simulink library "adi_ad9361_models"  (R2019b)
settings: Solver=VariableStepAuto  StartTime=0.0  StopTime=10.0  RelTol=1e-3
undefined symbols (not defined in the file): ad9361_preload, D, dBval, DCLeak_Matrix, designMultirateFIR, errordlg, fuzz_val, GainImb_Matrix, IP2_Matrix, IP3_Matrix, magnitude
libraries: simrfV2elements x20, simrfV2util1 x10, dsparch4 x8, simrfV2junction1 x8, simulink x8, dspmlti4 x6, ad9361_private x4, simulink_extras x2, dspsigattribs x2, simrfV2sources1 x2, simrfV2_lib x2, dspmathops x2
(part 1 of 2)
settings Model: Creator=gzucchel  LastModifiedBy=bhisma
settings SolverCC: MinimalZcImpactIntegration=on
settings DataIOCC: ReturnWorkspaceOutputs=off
settings DebuggingCC: PregeneratedLibrarySubsystemCodeDiagnostic=none  ArithmeticOperatorsInVariantConditions=warning
settings SFSimCC: SimUseLocalCustomCode=off  CustomCodeUndefinedFunction=UseInterfaceOnly
settings RTWCC: RTWUseLocalCustomCode=off
settings CodeAppCC: StateflowObjectComments=on

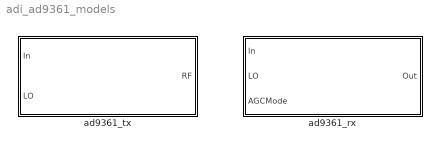
== system adi_ad9361_models ==
  ad9361_rx : Subsystem  LoadFcn=ad9361_preload(bdroot,'rx')  mask(ad9361_RX){TestSignal=Custom, LO=5200000000, RF=5200000000, Trf=5e-08/2, RF_BW=40, IQ_rate=40}
      mask prompts: TestSignal "Filter Configuration:"; LO "LO Frequency (Hz)"; RF "RF Center Frequency (Hz)"; Trf "Step Size RF Simulation (s)"; RF_BW "Input RF Bandwidth (MHz)"; IQ_rate "I/Q Sample Rate (MHz)"
      mask help: Model an Analog Devices ad9361 RF Receiver.
      mask init:
      | %load ad9361_rx_tables;
      | [ADIGainTable, ADIPhaseTable, ...
      |     DCLeak_Matrix, GainImb_Matrix, ...
      |     IP2_Matrix, IP3_Matrix] = ad9361_rx_gaintable(LO);
      | ad9361_rx_pars = ad9361_rx_initfcn(gcb,'Init');
      | ad9361_rx_pars = ad9361_rx_initfcn(gcb,'Build');
      mask Help:
      | Model an Analog Devices ad9361 RF Receiver. This model predicts thermal noise, spectral growth, LO carrier leakage and image signals, quantization noise in manual and slow attack control mode.
      | 
      | To change the automatic gain control mode, toggle the manual switch between manual mode and slow-attack control mode under the receiver mask. For manual mode, directly specify the index of the gain table in the constant block "manual index".
      | 
      | For signals with LTE 5MHz, LTE 10 MHz and LTE 20 MHz characteristics, the default configurations recommended by Analog Devices are directly available.
      | 
      | The filters are programmable. Use the Analog Devices Wizard App to custom design Filters. Select the option Custom in the Filter Configuration menu and click Design Filter button. The Filter Design app will open automatically. Make sure a receiver filter is designed instead of a transmitter filter. After designing the filter, click the button Export to Workspace in the App. The custom filter design is saved in the model set up. Next time a simulation is setup with custom filter configuration, the latest filter design is used.
      | 
      | Make sure that the input signal sample time and the expected step size of the RF simulation are the same. In case of a mismatch, an error is generated.
      mask TypeOptions TestSignal: 5MHz LTE | 10MHz LTE | 20MHz LTE | Custom
      mask Callback TestSignal:
      | % Set Mask visibilites and enables
      | ad9361_rx_mask_callbacks(gcb,'TestSignal')
      mask Callback Trf:
      | % block = gcb;
      | % p = Simulink.Mask.get(block);
      | % tmp = num2str(1/eval(get_param(gcb,'Trf'))/1e6,6);
      | % p.Parameters(5).Value = tmp;
      | set_param(gcb,'RF_BW',num2str(1/eval(get_param(gcb,'Trf'))/1e6,6));
      mask DialogControl ParameterGroupVar Prompt: ad9361 Receiver
      mask DialogControl Control2 Prompt: SpacerDesign
      mask DialogControl DesignFilter Prompt: Design Filter
      mask DialogControl DesignFilter Callback: ad9361_rx_initfcn(gcb,'DesignFilter');
      mask Display: text(0.5,0.5,'ad9361_RX','horizontalAlignment','center');
  ad9361_tx : Subsystem  LoadFcn=ad9361_preload(bdroot,'tx')  mask(ad9361_TX){TestSignal=5MHz LTE, LOFreq=2e9, Att=0, IQ_rate=7.68, RF_BW=122.88}
      mask prompts: TestSignal "Filter Configuration:"; LOFreq "LO Frequency (Hz)"; Att "Attenuation (dB)"; IQ_rate "I/Q Sample Rate (MHz)"; RF_BW "RF Bandwidth (MHz)"
      mask help: Model an Analog Devices ad9361 RF Transmitter.
      mask init:
      | ad9361_tx_pars = ad9361_tx_initfcn(gcb,'Init');
      | ad9361_tx_pars = ad9361_tx_initfcn(gcb,'Build');
      mask Help:
      | Model an Analog Devices ad9361 RF Transmitter. This predicts thermal noise, phase noise, spectral growth, LO carrier leakage and image signals.
      | 
      | To change the attenuation value, modify the constant value in Attenuation block under the Transmitter mask. Transmitter attenuation is tunable between 0 to 80dB in steps of 0.25dB.
      | 
      | For signals with LTE 5MHz, LTE 10 MHz and LTE 20 MHz characteristics, the default configurations recommended by Analog Devices are directly available.
      | 
      | The filters are programmable. Use the Analog Devices Wizard App to custom design Filters. Select the option Custom in the Filter Configuration menu and click Design Filter button. The Filter Design App will open automatically. Make sure a transmitter filter is designed instead of a receiver filter. After designing the filter, click the button Export to Workspace in the App. The custom filter design is saved in the model set up. Next time a simulation is setup with custom filter configuration, the latest filter design is used.
      | 
      | Make sure that the input signal sample time and the expected signal sample time are the same. In case of a mismatch, an error is generated.
      mask TypeOptions TestSignal: 5MHz LTE | 10MHz LTE | 20MHz LTE | Custom
      mask Callback TestSignal:
      | % Control DesignFilter visibility
      | ad9361_tx_mask_callbacks(gcb,'TestSignal')
      mask DialogControl ParameterGroupVar Prompt: ad9361 Transmitter
      mask DialogControl DesignFilter Prompt: Design Filter
      mask DialogControl DesignFilter Callback: [~] = ad9361_tx_initfcn(gcb,'DesignFilter');
      mask DialogControl Control3 Prompt: SpacerDesign
      mask Display: text(0.5,0.5,'ad9361_TX','horizontalAlignment','center');

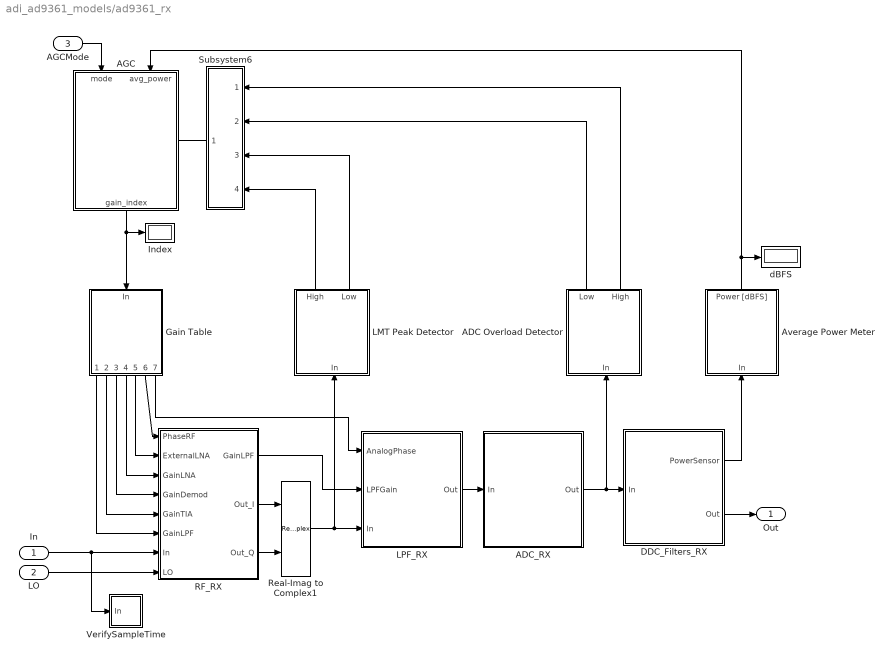
== system adi_ad9361_models/ad9361_rx ==
  In : Inport
  LO : Inport  Port=2
  AGCMode : Inport  Port=3
  ADC Overload Detector : Subsystem  mask{Ncycles=4, Lthreshold=47, Hthreshold=58}
      mask prompts: Ncycles "Number of Integration Cycles"; Lthreshold "Low Threshold"; Hthreshold "High Threshold"
      mask DialogControl DescGroupVar Prompt: ADC Overload Detector
  ADC_RX : Subsystem
  AGC : Stateflow chart  TreatAsAtomicUnit=on  mask{T=1, PeakOverLoadWait=1, SettlingDelay=32, FIR_Ts=ad9361_rx_pars.Tadc*ad9361_rx_pars.HB_interp, LMT_G_dec_fast=2, ADC_G_dec_fast=2, AGC_G_dec_fast=1, AGC_G_dec_slow=1, AGC_G_inc_fast=1, AGC_G_inc_slow=1, ManualGainIndex=76, C=3072 %approx 0.2ms, N_LMT_H=10, N_LMT_L=10, N_ADC_H=10, N_ADC_L=10, PT_HH=-8, PT_H=-10, PT_L=-12, PT_LL=-15, AGC_lock_level=-10, Max_Increase=5, EnableIncrGain=1, EnableGainIncAfterLock=1, AGC_attack_delay=10, EnergyDetectCount=32, IncrTime=5, LowPower=-13, PostLockStepSize=1, PowerMeasDuration=64, GainReset=No Gain Change, GainOffset=5, EnergyLost=1, StrongerSignalThreshold=10, GainLockExitCount=8, Overrange=8}
      mask prompts: T "Extra delay margin [us]"; PeakOverLoadWait "Peak Overload Wait Time [cycles]"; SettlingDelay "Settling Delay Power Meter [cycles]"; FIR_Ts "FIR Input Clock Time"; LMT_G_dec_fast "LMT peak large decrement"; ADC_G_dec_fast "ADC peak large decrement"; AGC_G_dec_fast "Average Power large decrement"; AGC_G_dec_slow "Average Power small decrement"; AGC_G_inc_fast "Average Power large increment"; AGC_G_inc_slow "Average Power small increment"; ManualGainIndex "Gain Index"; C "Gain Update Counter [cycles]"; N_LMT_H "LMT Upper Count"; N_LMT_L "LMT Lower Count"; N_ADC_H "ADC Upper Count"; N_ADC_L "ADC Lower Count"; PT_HH "Outer Threshold High [dBFS]"; PT_H "Inner Threshold High [dBFS]"; PT_L "Inner Threshold Low [dBFS]"; PT_LL "Outer Threshold Low [dBFS]"; AGC_lock_level "AGC Lock Level [dBFS]"; Max_Increase "AGC Lock Level Max Increase [Index]"; EnableIncrGain "Enable Gain Increment [0/1]"; EnableGainIncAfterLock "Enable Gain Increment After Gain Lock [0/1]"; AGC_attack_delay "Attack delay [us]"; EnergyDetectCount "Energy Detect Count [cycles]"; IncrTime "Increment Time [cycles]"; LowPower "Low Power Threshold"; PostLockStepSize "Post Lock Level Step Size [Index]"; PowerMeasDuration "Power Measurement Duration - State 5 [cycles]"; GainReset "Gain Index When Reset"; GainOffset "Optimize Gain Offset"; EnergyLost "Energy Lost Level [dB]"; StrongerSignalThreshold "Stronger Signal Threshold [dB]"; GainLockExitCount "Gain Lock Exit Count [cycles]"; Overrange "Overrange Count [Events]"
      mask init:
      | EnergyDetectCount = EnergyDetectCount*FIR_Ts;
      | C = C*FIR_Ts;
      | SettlingDelay = SettlingDelay*FIR_Ts;
      | PeakOverLoadWait = PeakOverLoadWait*FIR_Ts;
      | PowerMeasDuration = PowerMeasDuration*FIR_Ts;
      | IncrTime = IncrTime*FIR_Ts;
      | 
      | tmp = get_param(gcb,'parent');
      | n = get_param([tmp, '/Average Power Meter'], 'Ncycles');
      | DecPowerMeasDuration = str2num(n)*FIR_Ts;
  Average Power Meter : Subsystem  mask{Ncycles=64}
      mask prompts: Ncycles "Number of Integration Cycles"
      mask DialogControl DescGroupVar Prompt: Average Power Meter
  DDC_Filters_RX : Subsystem
  Gain Table : Subsystem
  "Index " : Display
  LMT Peak Detector : Subsystem  mask{HThreshold=800, LThreshold=704}
      mask prompts: HThreshold "High Threshold [mV]"; LThreshold "Low Threshold [mV]"
      mask DialogControl DescGroupVar Prompt: LMT Peak Detector
  LPF_RX : Subsystem
  RF_RX : Subsystem  mask{RF=RF, LO=LO, Tstep=Trf}
      mask prompts: RF "Center Frequency [Hz]"; LO "LO Frequency [Hz]"; Tstep "Sample Time [s]"
      mask init:
      | freq = [0.8e9, 2.4e9, 5.5e9];
      | nf   = [2,     3,     3.8];
      | NF   = interp1(freq, nf, LO,'linear','extrap');
      | 
      | if length(unique([RF LO])) == 2
      |     HB = [3 1];
      | else
      |     HB = 3;
      | end
      mask DialogControl DescGroupVar Prompt: ad9361 Receiver RF Front End
  Real-Imag to Complex1 : RealImagToComplex
  Subsystem6 : Subsystem  mask{NCyclesADC=4}
      mask prompts: NCyclesADC "ADC Integration Cycles"
  VerifySampleTime : Subsystem
  dBFS : Display
  Out : Outport  VectorParamsAs1DForOutWhenUnconnected=off
  wires:
  LO/1 -> RF_RX/8(LO)
  Gain Table/7(Analog phase) -> LPF_RX/1(AnalogPhase)
  ADC_RX/1(Out) -> DDC_Filters_RX/1(In), ADC Overload Detector/1(In)
  AGC/1(gain_index) -> "Index "/1, Gain Table/1(In)
  Average Power Meter/1(Power [dBFS]) -> AGC/2(avg_power), dBFS/1
  AGCMode/1 -> AGC/1(mode)
  Gain Table/5(External LNA) -> RF_RX/2(ExternalLNA)
  RF_RX/1("GainLPF ") -> LPF_RX/2(LPFGain)
  Subsystem6/1(Peak) -> AGC/Trigger
  In/1 -> VerifySampleTime/1(In), RF_RX/7(In)
  DDC_Filters_RX/2(Out) -> Out/1
  ADC Overload Detector/1(Low) -> Subsystem6/2(ADC_L)
  LMT Peak Detector/1(High) -> Subsystem6/4(LMT_H)
  ADC Overload Detector/2(High) -> Subsystem6/1(ADC_H)
  DDC_Filters_RX/1(PowerSensor) -> Average Power Meter/1(In)
  Gain Table/1(lpf) -> RF_RX/6(GainLPF)
  LMT Peak Detector/2(Low) -> Subsystem6/3(LMT_L)
  LPF_RX/1(Out) -> ADC_RX/1(In)
  Gain Table/4(lna) -> RF_RX/3(GainLNA)
  Gain Table/3(demod) -> RF_RX/4(GainDemod)
  Gain Table/2(tia) -> RF_RX/5(GainTIA)
  Real-Imag to Complex1/1 -> LPF_RX/3(In), LMT Peak Detector/1(In)
  RF_RX/3(Out_Q) -> Real-Imag to Complex1/2
  RF_RX/2(Out_I) -> Real-Imag to Complex1/1
  Gain Table/6(RF phase) -> RF_RX/1(PhaseRF)

== system adi_ad9361_models/ad9361_tx ==
  In : Inport
  LO : Inport  Port=2
  Analog_Filters_TX : Subsystem
  Attenuation : Constant  Value=Att
  DUC_Filters_TX : Subsystem
  RF_TX : Subsystem  mask{RF=LOFreq, Tstep=ad9361_tx_pars.Tduc}
      mask prompts: RF "Center Frequency (Hz)"; Tstep "Sample Time (s)"
      mask init:
      | Gain = interp1([800e6, 2.4e9, 5.5e9], [0, 0, -1]+8.3, RF, 'linear', 'extrap');
      | 
      | % Output referred IP3
      | oip3_800MHz = [23, 25, 10, 10];
      | oip3_2p4GHz = [19, 18,  6,  6];
      | oip3_5p5GHz = [17, 13,  2,  2];
      | Att_ip3     = [0 4 20 80];
      | if RF < 1.6e9
      |     OIP3v = oip3_800MHz;
      | elseif RF < 4e9
      |     OIP3v = oip3_2p4GHz;
      | else
      |     OIP3v = oip3_5p5GHz;
      | end
      | % Attenuation measurement data (dB)
      | Attdata  = [0  10  20  30  40  50   60   70   80];
      | % LO carrier leakage (dBm)
      | LO_leak  = ([-58 -52 -60 -71 -81 -82 -101 -102 -100]-Gain-6)/10;
      | % Gain imbalance (dBc)
      | Gain_imb = [-55.5 -66.2 -53.5 -57.5 -44.5 -46.3 -54.2 -46.1 -34.3]/20;
      | % Thermal noise floor (dBm/Hz)
      | NF       = interp1([800e6, 2.4e9, 5.5e9], [17, 18, 22.5], RF, 'linear', 'extrap');
      | 
      | set_param([gcb '/Configuration'], 'AddNoise','on');
      mask DialogControl Container1 Prompt: ad9361 Transmitter RF Front End
  VerifySampleTime : Subsystem
  RF : Outport  VectorParamsAs1DForOutWhenUnconnected=off
  wires:
  LO/1 -> RF_TX/4(LO)
  RF_TX/1(Out) -> RF/1
  DUC_Filters_TX/1(Out) -> Analog_Filters_TX/1(In)
  Attenuation/1 -> RF_TX/3(Attenuation)
  In/1 -> DUC_Filters_TX/1(In), VerifySampleTime/1(In)
  Analog_Filters_TX/2(Imaginary) -> RF_TX/2(In_Q)
  Analog_Filters_TX/1(Real) -> RF_TX/1(In_I)

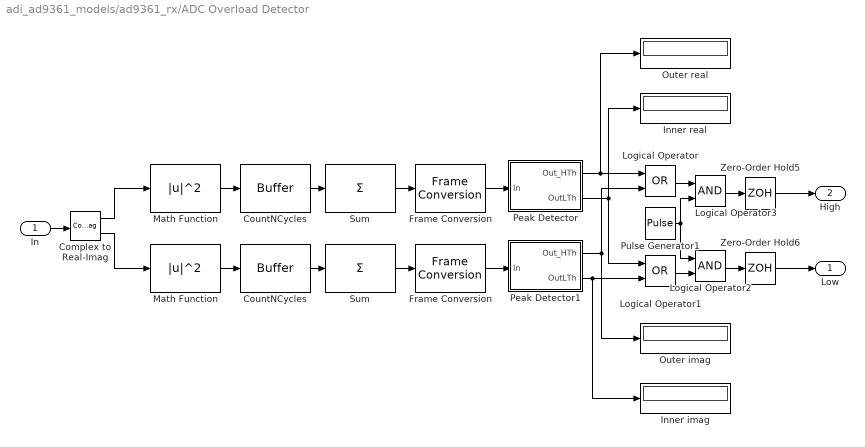
== system adi_ad9361_models/ad9361_rx/ADC Overload Detector ==
  In : Inport
  Complex to Real-Imag : ComplexToRealImag
  CountNCycles : Buffer  N=Ncycles
  "CountNCycles " : Buffer  N=Ncycles
  Frame Conversion : FrameConversion  OutFrame=Sample-based
  "Frame Conversion " : FrameConversion  OutFrame=Sample-based
  Inner imag : Display
  Inner real : Display
  Logical Operator : Logic  Operator=OR  AllPortsSameDT=off  OutDataTypeStr=boolean
  Logical Operator1 : Logic  Operator=OR  AllPortsSameDT=off  OutDataTypeStr=boolean
  Logical Operator2 : Logic  AllPortsSameDT=off  OutDataTypeStr=boolean
  Logical Operator3 : Logic  AllPortsSameDT=off  OutDataTypeStr=boolean
  Math Function : Math  Operator=magnitude^2  SaturateOnIntegerOverflow=on
  "Math Function " : Math  Operator=magnitude^2  SaturateOnIntegerOverflow=on
  Outer imag : Display
  Outer real : Display
  Peak Detector : Subsystem  mask{HThreshold=Hthreshold, LThreshold=Lthreshold}
      mask prompts: HThreshold "High Threshold (bit string) <4:0>"; LThreshold "Low Threshold (bit string) <4:0>"
  Peak Detector1 : Subsystem  mask{HThreshold=Hthreshold, LThreshold=Lthreshold}
      mask prompts: HThreshold "High Threshold (bit string) <4:0>"; LThreshold "Low Threshold (bit string) <4:0>"
  Pulse Generator1 : DiscretePulseGenerator  SampleTime=ad9361_rx_pars.Tadc*Ncycles
  Sum : Sum  Inputs=+
  "Sum " : Sum  Inputs=+
  Zero-Order Hold5 : ZeroOrderHold  SampleTime=Trf
  Zero-Order Hold6 : ZeroOrderHold  SampleTime=Trf
  Low : Outport  VectorParamsAs1DForOutWhenUnconnected=off
  High : Outport  Port=2  VectorParamsAs1DForOutWhenUnconnected=off
  wires:
  Zero-Order Hold6/1 -> Low/1
  Zero-Order Hold5/1 -> High/1
  Pulse Generator1/1 -> Logical Operator3/2, Logical Operator2/1
  Logical Operator3/1 -> Zero-Order Hold5/1
  Logical Operator1/1 -> Logical Operator2/2
  Logical Operator2/1 -> Zero-Order Hold6/1
  Logical Operator/1 -> Logical Operator3/1
  Complex to Real-Imag/2 -> "Math Function "/1
  Complex to Real-Imag/1 -> Math Function/1
  Peak Detector1/2(OutLTh) -> Logical Operator1/2, Inner imag/1
  Peak Detector1/1(Out_HTh) -> Outer imag/1, Logical Operator/2
  Peak Detector/1(Out_HTh) -> Logical Operator/1, Outer real/1
  Peak Detector/2(OutLTh) -> Inner real/1, Logical Operator1/1
  "Frame Conversion "/1 -> Peak Detector1/1(In)
  "Sum "/1 -> "Frame Conversion "/1
  "CountNCycles "/1 -> "Sum "/1
  "Math Function "/1 -> "CountNCycles "/1
  In/1 -> Complex to Real-Imag/1
  Frame Conversion/1 -> Peak Detector/1(In)
  Sum/1 -> Frame Conversion/1
  CountNCycles/1 -> Sum/1
  Math Function/1 -> CountNCycles/1

== system adi_ad9361_models/ad9361_rx/ADC_RX ==
  In : Inport
  ADC_I : Subsystem
  ADC_Q : Subsystem
  Complex to Real-Imag1 : ComplexToRealImag
  Real-Imag to Complex : RealImagToComplex
  Out : Outport  VectorParamsAs1DForOutWhenUnconnected=off
  wires:
  ADC_Q/1(Out) -> Real-Imag to Complex/2
  ADC_I/1(Out) -> Real-Imag to Complex/1
  Real-Imag to Complex/1 -> Out/1
  In/1 -> Complex to Real-Imag1/1
  Complex to Real-Imag1/2 -> ADC_Q/1(In)
  Complex to Real-Imag1/1 -> ADC_I/1(In)

== system adi_ad9361_models/ad9361_rx/Average Power Meter ==
  In : Inport
  Max saturation power dBm : Constant  Value=20*log10(4)+30
  Quantizer : Quantizer
  RMS : Subsystem
  Saturation : Saturate  UpperLimit=0  LowerLimit=-63.5
  Subtract : Sum  Inputs=+-
  dB Conversion : Subsystem  mask(dB Conversion){dBtype=dBm, intype=Amplitude, R=1, fuzz=on}
      mask prompts: dBtype "Convert to:"; intype "Input signal:"; R "Load resistance (ohms):"; fuzz "Add eps to input to protect against  "log(0) = -inf""
      mask help: Convert input of watts or volts to decibels. Voltage inputs are first converted to power relative to the specified load resistance, where P = (V^2)/R. When converting to dB, the reference power is 1 W. When converting to dBm, the reference power is 1 mW.
      mask init:
      | [str fuzz_val dBval] = dspblkdb2('init');
      | dspblkdb2('checkparam');
      | dspblkdb2('update');
      mask Help: eval('blocksethelp');
      mask TypeOptions dBtype: dB | dBm
      mask Callback dBtype: dspblkdb2
      mask TypeOptions intype: Power | Amplitude
      mask Callback intype: dspblkdb2
      mask Display: disp(str)
  Power [dBFS] : Outport  VectorParamsAs1DForOutWhenUnconnected=off
  wires:
  Saturation/1 -> Power [dBFS]/1
  RMS/1(Out) -> dB Conversion/1(in)
  In/1 -> RMS/1(In)
  dB Conversion/1(out) -> Subtract/1
  Quantizer/1 -> Saturation/1
  Subtract/1 -> Quantizer/1
  Max saturation power dBm/1 -> Subtract/2

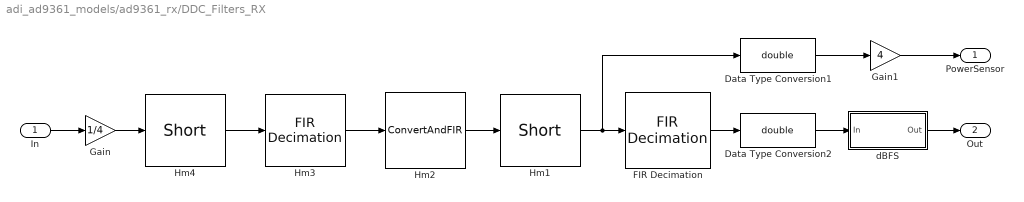
== system adi_ad9361_models/ad9361_rx/DDC_Filters_RX ==
  In : Inport
  Data Type Conversion1 : DataTypeConversion  OutDataTypeStr=double
  Data Type Conversion2 : DataTypeConversion  OutDataTypeStr=double
  FIR Decimation : dspmlti4/FIR Decimation  FilterSource=Filter object  h=fir1(35,0.4)  D=2  filtStruct=Direct form  FilterObject=ad9361_rx_pars.Hmd_rx  framing=Allow multirate processing  inputOffset=0  outputBufInitCond=0  roundingMode=Floor  overflowMode=off  firstCoeffDataTypeStr=Inherit: Same word length as input  firstCoeffMin=[]  firstCoeffMax=[]  firstCoeffLastDataTypeStr=Inherit: Same word length as input  outputDataTypeStr=Inherit: Same as accumulator  outputMin=[]  outputMax=[]  outputLastDataTypeStr=Inherit: Same as accumulator
  Gain : Gain  Gain=1/4
  Gain1 : Gain  Gain=4
  Hm1 : ad9361_private/Short  SystemSampleTime=-1  VariantControl=ad9361_tx_hm1Filt==0
      settings: SourceProductName=RF Blockset Models for Analog Devices RF Transceivers  SourceProductBaseCode=SIM_RF_TRANS
  Hm2 : ad9361_private/ConvertAndFIR  DataTypeOut=fixdt(1,16,14)  FilterObj=ad9361_rx_pars.Hm2_rx
      settings: SourceProductName=RF Blockset Models for Analog Devices RF Transceivers  SourceProductBaseCode=SIM_RF_TRANS
  Hm3 : dspmlti4/FIR Decimation  FilterSource=Filter object  h=designMultirateFIR(1,2)  D=2  filtStruct=Direct form  FilterObject=ad9361_rx_pars.Hm3_rx  framing=Enforce single-rate processing  inputOffset=0  outputBufInitCond=0  roundingMode=Floor  overflowMode=off  firstCoeffDataTypeStr=Inherit: Same word length as input  firstCoeffMin=[]  firstCoeffMax=[]  firstCoeffLastDataTypeStr=Inherit: Same word length as input  outputDataTypeStr=Inherit: Same as accumulator  outputMin=[]  outputMax=[]  outputLastDataTypeStr=Inherit: Same as accumulator
  Hm4 : ad9361_private/Short  SystemSampleTime=-1  VariantControl=ad9361_tx_hm1Filt==0
      settings: SourceProductName=RF Blockset Models for Analog Devices RF Transceivers  SourceProductBaseCode=SIM_RF_TRANS
  dBFS : Subsystem
  PowerSensor : Outport  VectorParamsAs1DForOutWhenUnconnected=off
  Out : Outport  Port=2  VectorParamsAs1DForOutWhenUnconnected=off
  wires:
  dBFS/1(Out) -> Out/1
  Data Type Conversion2/1 -> dBFS/1(In)
  Hm1/1 -> Data Type Conversion1/1, FIR Decimation/1
  Gain1/1 -> PowerSensor/1
  Data Type Conversion1/1 -> Gain1/1
  Gain/1 -> Hm4/1
  FIR Decimation/1 -> Data Type Conversion2/1
  Hm2/1 -> Hm1/1
  Hm3/1 -> Hm2/1
  Hm4/1 -> Hm3/1
  In/1 -> Gain/1

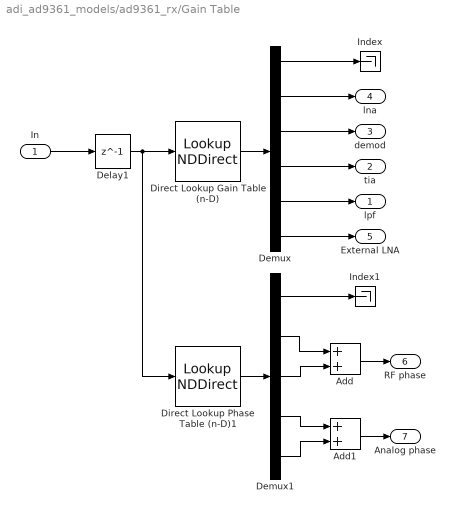
== system adi_ad9361_models/ad9361_rx/Gain Table ==
  In : Inport
  Add : Sum
  Add1 : Sum
  Delay1 : Delay  DelayLength=1  InitialCondition=76  SampleTime=Trf
  Demux : Demux  Outputs=6
  Demux1 : Demux  Outputs=5
  Direct Lookup Gain Table (n-D) : LookupNDDirect  InputsSelectThisObjectFromTable=Vector  Table=ADIGainTable'
  Direct Lookup Phase Table (n-D)1 : LookupNDDirect  InputsSelectThisObjectFromTable=Vector  Table=ADIPhaseTable'
  Index : Terminator
  Index1 : Terminator
  lpf : Outport  VectorParamsAs1DForOutWhenUnconnected=off
  tia : Outport  Port=2  VectorParamsAs1DForOutWhenUnconnected=off
  demod : Outport  Port=3  VectorParamsAs1DForOutWhenUnconnected=off
  lna : Outport  Port=4  VectorParamsAs1DForOutWhenUnconnected=off
  External LNA : Outport  Port=5  VectorParamsAs1DForOutWhenUnconnected=off
  RF phase : Outport  Port=6  VectorParamsAs1DForOutWhenUnconnected=off
  Analog phase : Outport  Port=7  VectorParamsAs1DForOutWhenUnconnected=off
  wires:
  Add1/1 -> Analog phase/1
  Add/1 -> RF phase/1
  Demux1/5 -> Add1/2
  Demux1/4 -> Add1/1
  Demux1/3 -> Add/2
  Demux1/2 -> Add/1
  Demux1/1 -> Index1/1
  Direct Lookup Phase Table (n-D)1/1 -> Demux1/1
  Demux/1 -> Index/1
  Demux/6 -> External LNA/1
  Direct Lookup Gain Table (n-D)/1 -> Demux/1
  Delay1/1 -> Direct Lookup Gain Table (n-D)/1, Direct Lookup Phase Table (n-D)1/1
  In/1 -> Delay1/1
  Demux/5 -> lpf/1
  Demux/4 -> tia/1
  Demux/2 -> lna/1
  Demux/3 -> demod/1

== system adi_ad9361_models/ad9361_rx/LMT Peak Detector ==
  In : Inport
  Abs : Abs
  HTh : Constant  Value=HThreshold*1e-3
  "High " : Display
  HighThreshold : RelationalOperator  OutDataTypeStr=boolean  RndMeth=Nearest
  LTh : Constant  Value=LThreshold*1e-3
  Logical Operator : Logic  AllPortsSameDT=off  OutDataTypeStr=boolean
  Logical Operator1 : Logic  AllPortsSameDT=off  OutDataTypeStr=boolean
  "Low " : Display
  LowThreshold : RelationalOperator  OutDataTypeStr=boolean  RndMeth=Nearest
  Pulse Generator2 : DiscretePulseGenerator  SampleTime=Trf
  High : Outport  SampleTime=Trf  VectorParamsAs1DForOutWhenUnconnected=off
  Low : Outport  Port=2  SampleTime=Trf  VectorParamsAs1DForOutWhenUnconnected=off
  wires:
  Logical Operator/1 -> Low/1
  Logical Operator1/1 -> High/1
  Pulse Generator2/1 -> Logical Operator/1, Logical Operator1/2
  LowThreshold/1 -> "Low "/1, Logical Operator/2
  HighThreshold/1 -> "High "/1, Logical Operator1/1
  In/1 -> Abs/1
  HTh/1 -> HighThreshold/2
  Abs/1 -> LowThreshold/1, HighThreshold/1
  LTh/1 -> LowThreshold/2

== system adi_ad9361_models/ad9361_rx/LPF_RX ==
  AnalogPhase : Inport
  LPFGain : Inport  Port=2
  In : Inport  Port=3
  Complex Phase Shift : commutil2/Complex Phase Shift
      settings: SourceProductName=Communications Toolbox  SourceProductBaseCode=CM
  Complex to Real-Imag : ComplexToRealImag
  Gain : Product
  LPF_I : dsparch4/Analog Filter Design  method=Butterworth  filttype=Lowpass  N=3  Wlo=1.4*ad9361_rx_pars.Fpass*2*pi  Whi=80  Rp=2  Rs=40
  "LPF_Q " : dsparch4/Analog Filter Design  method=Butterworth  filttype=Lowpass  N=3  Wlo=1.4*ad9361_rx_pars.Fpass*2*pi  Whi=80  Rp=2  Rs=40
  Phase[deg] : Display
  Real-Imag to Complex1 : RealImagToComplex
  ToRadians : Gain  Gain=pi/180
  dB2lin : Subsystem
  Out : Outport  VectorParamsAs1DForOutWhenUnconnected=off
  wires:
  ToRadians/1 -> Complex Phase Shift/2
  AnalogPhase/1 -> ToRadians/1, Phase[deg]/1
  In/1 -> Complex Phase Shift/1
  Complex to Real-Imag/2 -> "LPF_Q "/1
  LPF_I/1 -> Real-Imag to Complex1/1
  "LPF_Q "/1 -> Real-Imag to Complex1/2
  dB2lin/1(Out) -> Gain/1
  Gain/1 -> Complex to Real-Imag/1
  LPFGain/1 -> dB2lin/1(In)
  Complex Phase Shift/1 -> Gain/2
  Real-Imag to Complex1/1 -> Out/1
  Complex to Real-Imag/1 -> LPF_I/1

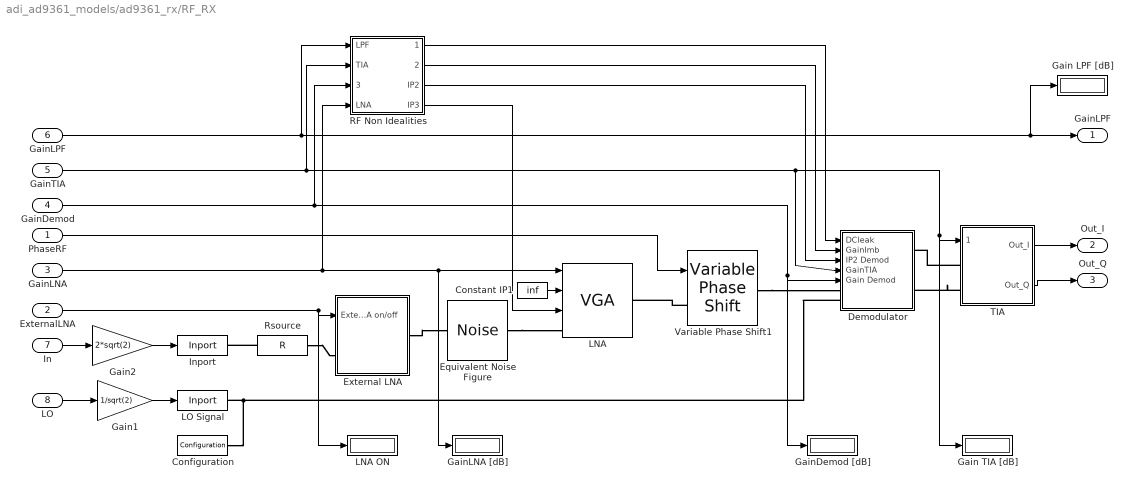
== system adi_ad9361_models/ad9361_rx/RF_RX ==
  PhaseRF : Inport
  ExternalLNA : Inport  Port=2
  GainLNA : Inport  Port=3
  GainDemod : Inport  Port=4
  GainTIA : Inport  Port=5
  GainLPF : Inport  Port=6
  In : Inport  Port=7
  LO : Inport  Port=8
  Configuration : simrfV2util1/Configuration  AutoFreq=off  Tones=unique([RF LO]) Hz  Harmonics=HB  NormalizeCarrierPower=on  SolverType=Auto  UseCCode=on  StepSize=Tstep s  AddNoise=on  defaultRNG=on  Seed=0  Temperature=290.0 K  SolverDelFlag=0  AbsTol=1e-6  RelTol=1e-3  MaxIter=10  ErrorEstimationType=2-norm over all variables  EnableInterpFilter=off  HiddenFIRfilterControllerParam=off  SmallSignalApprox=off  AllSimFreqs=on  SimFreqs=[] Hz  SimFreqsInternal=[]
      settings: SourceProductName=RF Blockset  SourceProductBaseCode=RB
  Constant IP1 : Constant  Value=inf
  Demodulator : Subsystem
  Equivalent Noise Figure : simrfV2sources1/Noise  SimulinkInputSignalType=Ideal voltage  NoiseType=White  NoisePSD=4*1.381e-23*290*50*10^(NF/10)  CarrierFreq=fc_RF Hz  AutoImpulseLength=on  ImpulseLength=1e-10 s  InternalGrounding=off
      settings: SourceProductName=RF Blockset  SourceProductBaseCode=RB
  External LNA : Subsystem
  Gain LPF [dB] : Display
  Gain TIA [dB] : Display
  Gain1 : Gain  Gain=1/sqrt(2)
  Gain2 : Gain  Gain=2*sqrt(2)
  GainDemod [dB] : Display
  GainLNA [dB] : Display
  Inport : simrfV2util1/Inport  SimulinkInputSignalType=Ideal voltage  CarrierFreq=RF Hz  ZS=0  InternalGrounding=on
      settings: SourceProductName=RF Blockset  SourceProductBaseCode=RB
  LNA : simrfV2elements/VGA  classname=vga  Zin=50  Zout=50  IO=Input  InternalGrounding=on
      settings: SourceProductName=RF Blockset  SourceProductBaseCode=RB
  LNA ON : Display
  LO Signal : simrfV2util1/Inport  SimulinkInputSignalType=Ideal voltage  CarrierFreq=LO Hz  ZS=0  InternalGrounding=on
      settings: SourceProductName=RF Blockset  SourceProductBaseCode=RB
  RF Non Idealities : Subsystem
  Rsource : simrfV2elements/R  classname=resistor  Resistance=50 Ohm  AddNoise=on
      settings: SourceProductName=RF Blockset  SourceProductBaseCode=RB
  TIA : Subsystem
  Variable Phase Shift1 : simrfV2elements/Variable Phase Shift  classname=varphase  PhaseShift_unit=deg  SparamZ0=50  InternalGrounding=on
      settings: SourceProductName=RF Blockset  SourceProductBaseCode=RB
  "GainLPF " : Outport  VectorParamsAs1DForOutWhenUnconnected=off
  Out_I : Outport  Port=2  VectorParamsAs1DForOutWhenUnconnected=off
  Out_Q : Outport  Port=3  VectorParamsAs1DForOutWhenUnconnected=off
  wires:
  Gain1/1 -> LO Signal/1
  LO/1 -> Gain1/1
  PhaseRF/1 -> Variable Phase Shift1/1
  TIA/2(Out_Q) -> Out_Q/1
  RF Non Idealities/2(GainImbalance) -> Demodulator/2(GainImb)
  ExternalLNA/1 -> External LNA/1(ExternalLNA on/off), LNA ON/1
  Constant IP1/1 -> LNA/2
  RF Non Idealities/4(IP3) -> LNA/3
  RF Non Idealities/3(IP2) -> Demodulator/3(IP2 Demod)
  RF Non Idealities/1(DCLeakage) -> Demodulator/1(DCleak)
  GainLNA/1 -> GainLNA [dB]/1, LNA/1, RF Non Idealities/4(LNA)
  GainDemod/1 -> RF Non Idealities/3(Demod), GainDemod [dB]/1, Demodulator/5(Gain Demod)
  GainTIA/1 -> RF Non Idealities/2(TIA), TIA/1(Gain TIA), Gain TIA [dB]/1, Demodulator/4(GainTIA)
  GainLPF/1 -> RF Non Idealities/1(LPF), Gain LPF [dB]/1, "GainLPF "/1
  TIA/1(Out_I) -> Out_I/1
  Gain2/1 -> Inport/1
  In/1 -> Gain2/1
  connections:
  Variable Phase Shift1/RConn1 -- Demodulator/LConn1
  Variable Phase Shift1/LConn1 -- LNA/RConn1
  Demodulator/LConn2 -- Configuration/LConn1 -- LO Signal/RConn1
  External LNA/RConn1 -- Equivalent Noise Figure/RConn1
  Rsource/LConn1 -- External LNA/LConn1
  TIA/LConn1 -- Demodulator/RConn1
  TIA/LConn2 -- Demodulator/RConn2
  Equivalent Noise Figure/LConn1 -- LNA/LConn1
  Rsource/RConn1 -- Inport/RConn1

== system adi_ad9361_models/ad9361_rx/Subsystem6 ==
  ADC_H : Inport
  ADC_L : Inport  Port=2
  LMT_L : Inport  Port=3
  LMT_H : Inport  Port=4
  Data Type Conversion : DataTypeConversion  OutDataTypeStr=boolean
  Logical Operator : Logic  Operator=OR  AllPortsSameDT=off  OutDataTypeStr=boolean
  Mux : Mux  Inputs=5
  Subsystem1 : Subsystem
  Wblk5 : Subsystem
  Wblk6 : Subsystem
  Wblk7 : Subsystem
  Peak : Outport  VectorParamsAs1DForOutWhenUnconnected=off
  wires:
  Mux/1 -> Peak/1
  LMT_H/1 -> Logical Operator/2, Mux/4, Wblk5/2(Sin)  "LMT_H"
  ADC_H/1 -> Wblk5/1(Win)
  ADC_L/1 -> Wblk6/1(Win)
  Data Type Conversion/1 -> Mux/5  "Event"
  Subsystem1/1(START) -> Data Type Conversion/1
  Wblk5/1(Wout) -> Logical Operator/1, Mux/1  "ADC_H"
  Wblk6/1(Wout) -> Mux/2  "ADC_L"
  Wblk7/1(Wout) -> Mux/3  "LMT_L"
  Logical Operator/1 -> Wblk6/2(Sin), Wblk7/2(Sin)
  LMT_L/1 -> Wblk7/1(Win)

== system adi_ad9361_models/ad9361_rx/VerifySampleTime ==
  In : Inport
  Abs : Abs
  Assertion : Assertion  AssertionFailFcn=errordlg('Test signal sample time and RF simulation step size are not consistent');
  Compare To Constant : simulink/Logic and Bit Operations/Compare To Constant  relop=<=  const=eps(1/Trf)  OutDataTypeStr=boolean
  Constant : Constant  Value=Trf
  Subtract : Sum  Inputs=+-
  Weighted Sample Time : SampleTimeMath  TsampMathOp=Ts Only
  wires:
  In/1 -> Weighted Sample Time/1
  Weighted Sample Time/1 -> Subtract/1
  Constant/1 -> Subtract/2
  Subtract/1 -> Abs/1
  Abs/1 -> Compare To Constant/1
  Compare To Constant/1 -> Assertion/1

== system adi_ad9361_models/ad9361_tx/Analog_Filters_TX ==
  In : Inport
  " AnalogFilter " : dsparch4/Analog Filter Design  method=Butterworth  filttype=Lowpass  N=3  Wlo=1.6*ad9361_tx_pars.Fpass*2*pi  Whi=80  Rp=2  Rs=40
  AnalogFilter : dsparch4/Analog Filter Design  method=Butterworth  filttype=Lowpass  N=3  Wlo=1.6*ad9361_tx_pars.Fpass*2*pi  Whi=80  Rp=2  Rs=40
  "AnalogFilter " : dsparch4/Analog Filter Design  method=Butterworth  filttype=Lowpass  N=1  Wlo=5*ad9361_tx_pars.Fpass*2*pi  Whi=80  Rp=2  Rs=40
  AnalogFilters : dsparch4/Analog Filter Design  method=Butterworth  filttype=Lowpass  N=1  Wlo=5*ad9361_tx_pars.Fpass*2*pi  Whi=80  Rp=2  Rs=40
  Complex to Real-Imag : ComplexToRealImag
  Real : Outport  VectorParamsAs1DForOutWhenUnconnected=off
  Imaginary : Outport  Port=2  VectorParamsAs1DForOutWhenUnconnected=off
  wires:
  AnalogFilters/1 -> Imaginary/1
  Complex to Real-Imag/1 -> AnalogFilter/1
  In/1 -> Complex to Real-Imag/1
  Complex to Real-Imag/2 -> " AnalogFilter "/1
  AnalogFilter/1 -> "AnalogFilter "/1
  " AnalogFilter "/1 -> AnalogFilters/1
  "AnalogFilter "/1 -> Real/1

== system adi_ad9361_models/ad9361_tx/DUC_Filters_TX ==
  In : Inport
  Add : Sum
  Band-Limited White Noise : simulink/Sources/Band-Limited White Noise  Cov=[0.1]  Ts=ad9361_tx_pars.Tduc  seed=[23341]
  Hm1 : dspmlti4/FIR Interpolation  FilterSource=Filter object  h=designMultirateFIR(3,1)  L=3  FilterObject=ad9361_tx_pars.Hm1_tx  framing=Enforce single-rate processing  outputBufInitCond=0  roundingMode=Floor  overflowMode=off  firstCoeffDataTypeStr=Inherit: Same word length as input  firstCoeffMin=[]  firstCoeffMax=[]  firstCoeffLastDataTypeStr=Inherit: Same word length as input  outputDataTypeStr=Inherit: Same as accumulator  outputMin=[]  outputMax=[]  outputLastDataTypeStr=Inherit: Same as accumulator
      settings: SourceProductName=DSP System Toolbox
  Hm2 : dspmlti4/FIR Interpolation  FilterSource=Filter object  h=designMultirateFIR(3,1)  L=3  FilterObject=ad9361_tx_pars.Hm2_tx  framing=Enforce single-rate processing  outputBufInitCond=0  roundingMode=Floor  overflowMode=off  firstCoeffDataTypeStr=Inherit: Same word length as input  firstCoeffMin=[]  firstCoeffMax=[]  firstCoeffLastDataTypeStr=Inherit: Same word length as input  outputDataTypeStr=Inherit: Same as accumulator  outputMin=[]  outputMax=[]  outputLastDataTypeStr=Inherit: Same as accumulator
      settings: SourceProductName=DSP System Toolbox
  Hm3 : dspmlti4/FIR Interpolation  FilterSource=Filter object  h=designMultirateFIR(3,1)  L=3  FilterObject=ad9361_tx_pars.Hm3_tx  framing=Enforce single-rate processing  outputBufInitCond=0  roundingMode=Floor  overflowMode=off  firstCoeffDataTypeStr=Inherit: Same word length as input  firstCoeffMin=[]  firstCoeffMax=[]  firstCoeffLastDataTypeStr=Inherit: Same word length as input  outputDataTypeStr=Inherit: Same as accumulator  outputMin=[]  outputMax=[]  outputLastDataTypeStr=Inherit: Same as accumulator
      settings: SourceProductName=DSP System Toolbox
  Hmd : dspmlti4/FIR Interpolation  FilterSource=Filter object  h=fir1(15,1/4)  L=3  FilterObject=ad9361_tx_pars.Hmd_tx  framing=Allow multirate processing  outputBufInitCond=0  roundingMode=Floor  overflowMode=off  firstCoeffDataTypeStr=Inherit: Same word length as input  firstCoeffMin=[]  firstCoeffMax=[]  firstCoeffLastDataTypeStr=Inherit: Same word length as input  outputDataTypeStr=Inherit: Same as accumulator  outputMin=[]  outputMax=[]  outputLastDataTypeStr=Inherit: Same as accumulator
      settings: SourceProductName=DSP System Toolbox
  NoiseFloor : dspmathops/dB Gain  dB=-130-20-8  intype=Amplitude
      settings: SourceProductName=DSP System Toolbox  SourceProductBaseCode=DS
  Short : ad9361_private/Short  SystemSampleTime=-1  VariantControl=ad9361_tx_hm1Filt==0
      settings: SourceProductName=RF Blockset Models for Analog Devices RF Transceivers  SourceProductBaseCode=SIM_RF_TRANS
  dB Gain : dspmathops/dB Gain  dB=log2(ad9361_tx_pars.BW_duc/ad9361_tx_pars.SamplingRate)*6  intype=Amplitude
      settings: SourceProductName=DSP System Toolbox  SourceProductBaseCode=DS
  Out : Outport  VectorParamsAs1DForOutWhenUnconnected=off
  wires:
  Hm2/1 -> Hm3/1
  Short/1 -> dB Gain/1
  NoiseFloor/1 -> Add/1
  Band-Limited White Noise/1 -> NoiseFloor/1
  Add/1 -> Out/1
  dB Gain/1 -> Add/2
  In/1 -> Hmd/1
  Hm3/1 -> Short/1
  Hm1/1 -> Hm2/1
  Hmd/1 -> Hm1/1

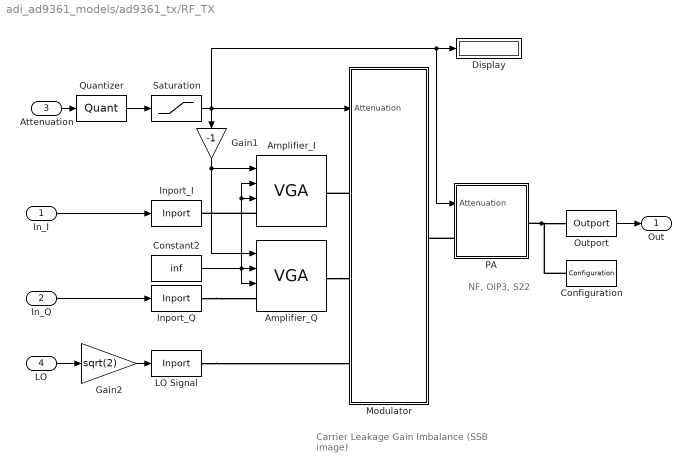
== system adi_ad9361_models/ad9361_tx/RF_TX ==
  note: Carrier Leakage
      | Gain Imbalance (SSB image)
  note: NF, OIP3, S22
  In_I : Inport
  In_Q : Inport  Port=2
  Attenuation : Inport  Port=3
  LO : Inport  Port=4
  Amplifier_I : simrfV2elements/VGA  classname=vga  Zin=50  Zout=50  IO=Output  InternalGrounding=on
      settings: SourceProductName=RF Blockset  SourceProductBaseCode=RB
  Amplifier_Q : simrfV2elements/VGA  classname=vga  Zin=50  Zout=50  IO=Output  InternalGrounding=on
      settings: SourceProductName=RF Blockset  SourceProductBaseCode=RB
  Configuration : simrfV2util1/Configuration  AutoFreq=off  Tones=RF Hz  Harmonics=3  NormalizeCarrierPower=on  SolverType=Auto  UseCCode=on  StepSize=Tstep s  AddNoise=on  defaultRNG=on  Seed=0  Temperature=290.0 K  SolverDelFlag=0  AbsTol=1e-6  RelTol=1e-3  MaxIter=10  ErrorEstimationType=2-norm over all variables  EnableInterpFilter=off  HiddenFIRfilterControllerParam=off  SmallSignalApprox=off  AllSimFreqs=on  SimFreqs=[] Hz  SimFreqsInternal=[]
      settings: SourceProductName=RF Blockset  SourceProductBaseCode=RB
  Constant2 : Constant  Value=inf
  Display : Display
      settings: Decimation=100
  Gain1 : Gain  Gain=-1
  Gain2 : Gain  Gain=sqrt(2)
  Inport_I : simrfV2util1/Inport  SimulinkInputSignalType=Power  CarrierFreq=0 Hz  ZS=50  InternalGrounding=on
      settings: SourceProductName=RF Blockset  SourceProductBaseCode=RB
  Inport_Q : simrfV2util1/Inport  SimulinkInputSignalType=Power  CarrierFreq=0 Hz  ZS=50  InternalGrounding=on
      settings: SourceProductName=RF Blockset  SourceProductBaseCode=RB
  LO Signal : simrfV2util1/Inport  SimulinkInputSignalType=Ideal voltage  CarrierFreq=LOFreq Hz  ZS=0  InternalGrounding=on
      settings: SourceProductName=RF Blockset  SourceProductBaseCode=RB
  Modulator : Subsystem
  Outport : simrfV2util1/Outport  SensorType=Power  OutputFormat=Complex Baseband  CarrierFreq=RF Hz  ZL=50  InternalGrounding=on  StepSize=-1 s  AutoStep=off
      settings: SourceProductName=RF Blockset  SourceProductBaseCode=RB
  PA : Subsystem
  Quantizer : Quantizer  QuantizationInterval=0.25
  Saturation : Saturate  UpperLimit=89.75  LowerLimit=0
  Out : Outport  VectorParamsAs1DForOutWhenUnconnected=off
  wires:
  Gain2/1 -> LO Signal/1
  LO/1 -> Gain2/1
  Gain1/1 -> Amplifier_Q/1, Amplifier_I/1
  Constant2/1 -> Amplifier_I/2, Amplifier_I/3, Amplifier_Q/2, Amplifier_Q/3
  Outport/1 -> Out/1
  Quantizer/1 -> Saturation/1
  Saturation/1 -> Display/1, PA/1(" Attenuation"), Modulator/1(Attenuation), Gain1/1
  Attenuation/1 -> Quantizer/1
  In_Q/1 -> Inport_Q/1
  In_I/1 -> Inport_I/1
  connections:
  LO Signal/RConn1 -- Modulator/LConn3
  Modulator/LConn1 -- Amplifier_I/RConn1
  PA/LConn1 -- Modulator/RConn1
  PA/RConn1 -- Outport/LConn1 -- Configuration/LConn1
  Amplifier_Q/RConn1 -- Modulator/LConn2
  Inport_Q/RConn1 -- Amplifier_Q/LConn1
  Amplifier_I/LConn1 -- Inport_I/RConn1

== system adi_ad9361_models/ad9361_tx/VerifySampleTime ==
  In : Inport
  Abs : Abs
  Assertion : Assertion  AssertionFailFcn=errordlg('Test signal sample time and I/Q sample rate are not consistent');
  Compare To Constant : simulink/Logic and Bit Operations/Compare To Constant  relop=<=  const=eps(1/ad9361_tx_pars.SamplingRate)*1e12  OutDataTypeStr=boolean
  Constant : Constant  Value=1/ad9361_tx_pars.SamplingRate
  Subtract : Sum  Inputs=+-
  Weighted Sample Time : SampleTimeMath  TsampMathOp=Ts Only
  wires:
  Compare To Constant/1 -> Assertion/1
  Subtract/1 -> Abs/1
  Constant/1 -> Subtract/2
  Weighted Sample Time/1 -> Subtract/1
  In/1 -> Weighted Sample Time/1
  Abs/1 -> Compare To Constant/1

== system adi_ad9361_models/ad9361_rx/ADC Overload Detector/Peak Detector ==
  In : Inport
  HTh : Constant  Value=Hthreshold  SampleTime=ad9361_rx_pars.Tadc*Ncycles
  HighThreshold : RelationalOperator  OutDataTypeStr=boolean  RndMeth=Nearest
  LTh : Constant  Value=Lthreshold  SampleTime=ad9361_rx_pars.Tadc*Ncycles
  LowThreshold : RelationalOperator  OutDataTypeStr=boolean  RndMeth=Nearest
  Out_HTh : Outport  VectorParamsAs1DForOutWhenUnconnected=off
  OutLTh : Outport  Port=2  VectorParamsAs1DForOutWhenUnconnected=off
  wires:
  HTh/1 -> HighThreshold/2
  In/1 -> LowThreshold/1, HighThreshold/1
  LTh/1 -> LowThreshold/2
  HighThreshold/1 -> Out_HTh/1
  LowThreshold/1 -> OutLTh/1

== system adi_ad9361_models/ad9361_rx/ADC Overload Detector/Peak Detector1 ==
  In : Inport
  HTh : Constant  Value=Hthreshold  SampleTime=ad9361_rx_pars.Tadc*Ncycles
  HighThreshold : RelationalOperator  OutDataTypeStr=boolean  RndMeth=Nearest
  LTh : Constant  Value=Lthreshold  SampleTime=ad9361_rx_pars.Tadc*Ncycles
  LowThreshold : RelationalOperator  OutDataTypeStr=boolean  RndMeth=Nearest
  Out_HTh : Outport  VectorParamsAs1DForOutWhenUnconnected=off
  OutLTh : Outport  Port=2  VectorParamsAs1DForOutWhenUnconnected=off
  wires:
  LowThreshold/1 -> OutLTh/1
  HighThreshold/1 -> Out_HTh/1
  LTh/1 -> LowThreshold/2
  In/1 -> HighThreshold/1, LowThreshold/1
  HTh/1 -> HighThreshold/2

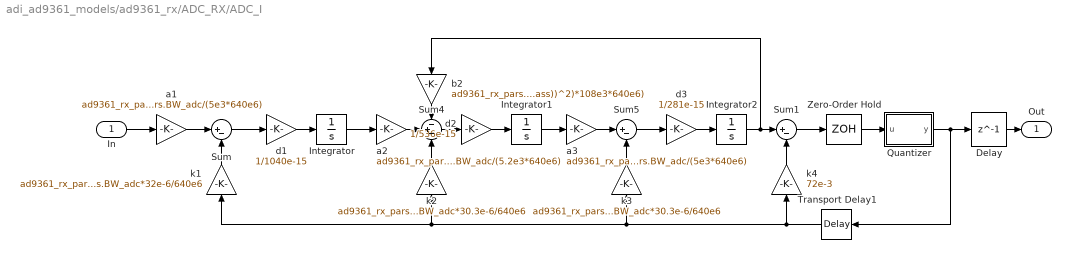
== system adi_ad9361_models/ad9361_rx/ADC_RX/ADC_I ==
  In : Inport
  Delay : Delay  DelayLength=1
  Integrator : Integrator  LimitOutput=on  UpperSaturationLimit=0.9  LowerSaturationLimit=-0.9
  Integrator1 : Integrator  LimitOutput=on  UpperSaturationLimit=0.9  LowerSaturationLimit=-0.9
  Integrator2 : Integrator  LimitOutput=on  UpperSaturationLimit=0.9  LowerSaturationLimit=-0.9
  Quantizer : Subsystem
  Sum : Sum  Inputs=|+-
  Sum1 : Sum  Inputs=|+-
  Sum4 : Sum  Inputs=-+-
  Sum5 : Sum  Inputs=|+-
  Transport Delay1 : TransportDelay  DelayTime=ad9361_rx_pars.Tadc/2
  Zero-Order Hold : ZeroOrderHold  SampleTime=ad9361_rx_pars.Tadc
  a1 : Gain  Gain=ad9361_rx_pars.BW_adc/(5e3*640e6)
  a2 : Gain  Gain=ad9361_rx_pars.BW_adc/(5.2e3*640e6)
  a3 : Gain  Gain=ad9361_rx_pars.BW_adc/(5e3*640e6)
  b2 : Gain  Gain=ad9361_rx_pars.BW_adc*1024/(4*((ad9361_rx_pars.BW_adc/(2*ad9361_rx_pars.Fpass))^2)*108e3*640e6)
  d1 : Gain  Gain=1/1040e-15
  d2 : Gain  Gain=1/536e-15
  d3 : Gain  Gain=1/281e-15
  k1 : Gain  Gain=ad9361_rx_pars.BW_adc*32e-6/640e6
  k2 : Gain  Gain=ad9361_rx_pars.BW_adc*30.3e-6/640e6
  k3 : Gain  Gain=ad9361_rx_pars.BW_adc*30.3e-6/640e6
  k4 : Gain  Gain=72e-3
  Out : Outport  VectorParamsAs1DForOutWhenUnconnected=off
  wires:
  Delay/1 -> Out/1
  Transport Delay1/1 -> k3/1, k2/1, k1/1, k4/1
  Quantizer/1(y) -> Delay/1, Transport Delay1/1
  k4/1 -> Sum1/2
  Sum1/1 -> Zero-Order Hold/1
  a3/1 -> Sum5/1
  b2/1 -> Sum4/1
  k3/1 -> Sum5/2
  k2/1 -> Sum4/3
  a2/1 -> Sum4/2
  Zero-Order Hold/1 -> Quantizer/1(u)
  Sum/1 -> d1/1
  Integrator/1 -> a2/1
  d1/1 -> Integrator/1
  Integrator1/1 -> a3/1
  d2/1 -> Integrator1/1
  Integrator2/1 -> b2/1, Sum1/1
  In/1 -> a1/1
  d3/1 -> Integrator2/1
  Sum4/1 -> d2/1
  Sum5/1 -> d3/1
  a1/1 -> Sum/1
  k1/1 -> Sum/2

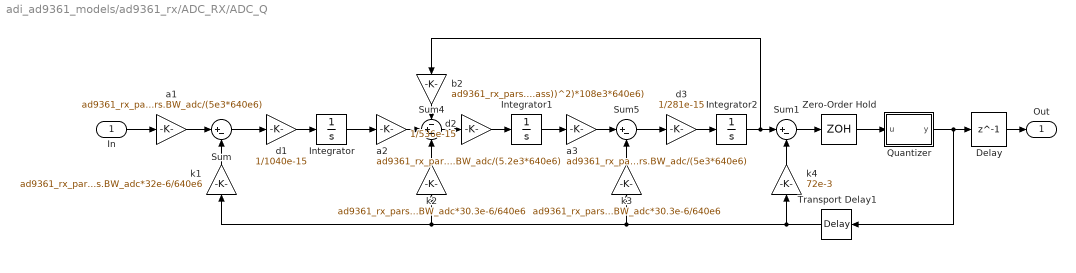
== system adi_ad9361_models/ad9361_rx/ADC_RX/ADC_Q ==
  In : Inport
  Delay : Delay  DelayLength=1
  Integrator : Integrator  LimitOutput=on  UpperSaturationLimit=0.9  LowerSaturationLimit=-0.9
  Integrator1 : Integrator  LimitOutput=on  UpperSaturationLimit=0.9  LowerSaturationLimit=-0.9
  Integrator2 : Integrator  LimitOutput=on  UpperSaturationLimit=0.9  LowerSaturationLimit=-0.9
  Quantizer : Subsystem
  Sum : Sum  Inputs=|+-
  Sum1 : Sum  Inputs=|+-
  Sum4 : Sum  Inputs=-+-
  Sum5 : Sum  Inputs=|+-
  Transport Delay1 : TransportDelay  DelayTime=ad9361_rx_pars.Tadc/2
  Zero-Order Hold : ZeroOrderHold  SampleTime=ad9361_rx_pars.Tadc
  a1 : Gain  Gain=ad9361_rx_pars.BW_adc/(5e3*640e6)
  a2 : Gain  Gain=ad9361_rx_pars.BW_adc/(5.2e3*640e6)
  a3 : Gain  Gain=ad9361_rx_pars.BW_adc/(5e3*640e6)
  b2 : Gain  Gain=ad9361_rx_pars.BW_adc*1024/(4*((ad9361_rx_pars.BW_adc/(2*ad9361_rx_pars.Fpass))^2)*108e3*640e6)
  d1 : Gain  Gain=1/1040e-15
  d2 : Gain  Gain=1/536e-15
  d3 : Gain  Gain=1/281e-15
  k1 : Gain  Gain=ad9361_rx_pars.BW_adc*32e-6/640e6
  k2 : Gain  Gain=ad9361_rx_pars.BW_adc*30.3e-6/640e6
  k3 : Gain  Gain=ad9361_rx_pars.BW_adc*30.3e-6/640e6
  k4 : Gain  Gain=72e-3
  Out : Outport  VectorParamsAs1DForOutWhenUnconnected=off
  wires:
  k1/1 -> Sum/2
  a1/1 -> Sum/1
  Sum5/1 -> d3/1
  Sum4/1 -> d2/1
  d3/1 -> Integrator2/1
  In/1 -> a1/1
  Integrator2/1 -> Sum1/1, b2/1
  d2/1 -> Integrator1/1
  Integrator1/1 -> a3/1
  d1/1 -> Integrator/1
  Integrator/1 -> a2/1
  Sum/1 -> d1/1
  Zero-Order Hold/1 -> Quantizer/1(u)
  a2/1 -> Sum4/2
  k2/1 -> Sum4/3
  k3/1 -> Sum5/2
  b2/1 -> Sum4/1
  a3/1 -> Sum5/1
  Sum1/1 -> Zero-Order Hold/1
  k4/1 -> Sum1/2
  Quantizer/1(y) -> Delay/1, Transport Delay1/1
  Transport Delay1/1 -> k4/1, k1/1, k2/1, k3/1
  Delay/1 -> Out/1

== system adi_ad9361_models/ad9361_rx/Average Power Meter/RMS ==
  In : Inport
  CountNCycles : Buffer  N=Ncycles
  Frame Conversion : FrameConversion  OutFrame=Sample-based
  Gain2 : Gain  Gain=1/Ncycles
  Root : Sqrt  SaturateOnIntegerOverflow=on
  Squared : Math  Operator=magnitude^2  SaturateOnIntegerOverflow=on
  Sum : Sum  Inputs=+
  Out : Outport  VectorParamsAs1DForOutWhenUnconnected=off
  wires:
  In/1 -> CountNCycles/1
  Gain2/1 -> Root/1
  Root/1 -> Frame Conversion/1
  Squared/1 -> Sum/1
  CountNCycles/1 -> Squared/1
  Frame Conversion/1 -> Out/1
  Sum/1 -> Gain2/1

== system adi_ad9361_models/ad9361_rx/Average Power Meter/dB Conversion ==
  in : Inport
  Constant : Constant  Value=fuzz_val  OutDataTypeStr=Inherit: Inherit via back propagation
  Constant1 : Constant  Value=dBval  OutDataTypeStr=Inherit: Inherit via back propagation
  Err if non-flt : dspsigattribs/Check Signal Attributes  SigAttribCheckMethod=Does not match attributes exactly  Complexity=Ignore  Frame=Ignore  DimsCheckMethod=Ignore  Dimensions=1-D  DatatypeCheckMethod=Is...  DatatypeGeneral=Floating-point  DtypeFloatSpecific=Any floating-point  DtypeFixedSpecific=Any fixed-point  DtypeIntSpecific=Any integer  SampleMode=Ignore
      settings: SourceProductName=DSP System Toolbox  SourceProductBaseCode=DS
  Error if Cplx : dspsigattribs/Check Signal Attributes  SigAttribCheckMethod=Matches attributes exactly  Complexity=Complex  Frame=Ignore  DimsCheckMethod=Ignore  Dimensions=1-D  DatatypeCheckMethod=Ignore  DatatypeGeneral=Boolean  DtypeFloatSpecific=Any floating-point  DtypeFixedSpecific=Any fixed-point  DtypeIntSpecific=Any integer  SampleMode=Ignore
      settings: SourceProductName=DSP System Toolbox  SourceProductBaseCode=DS
  Gain : Gain  Gain=10  SaturateOnIntegerOverflow=on  OutDataTypeStr=Inherit: Same as input  ParamDataTypeStr=Inherit: Same as input
  Magsq : Math  Operator=magnitude^2  SaturateOnIntegerOverflow=on
  Scale by R : Gain  Gain=1./R  SaturateOnIntegerOverflow=on  OutDataTypeStr=Inherit: Same as input  ParamDataTypeStr=Inherit: Same as input
  Sum1 : Sum  SaturateOnIntegerOverflow=on  InputSameDT=on  OutDataTypeStr=Inherit: Same as first input
  Sum2 : Sum  SaturateOnIntegerOverflow=on  InputSameDT=on  OutDataTypeStr=Inherit: Same as first input
  log10 : Math  Operator=log10  SaturateOnIntegerOverflow=on
  out : Outport  InitialOutput=0  VectorParamsAs1DForOutWhenUnconnected=off
  wires:
  Constant1/1 -> Sum2/2
  Sum2/1 -> out/1
  Gain/1 -> Sum2/1
  Constant/1 -> Sum1/2
  Sum1/1 -> Magsq/1
  Error if Cplx/1 -> Sum1/1
  in/1 -> Err if non-flt/1
  Err if non-flt/1 -> Error if Cplx/1
  Scale by R/1 -> log10/1
  Magsq/1 -> Scale by R/1
  log10/1 -> Gain/1

== system adi_ad9361_models/ad9361_rx/DDC_Filters_RX/dBFS ==
  In : Inport
  Complex to Real-Imag : ComplexToRealImag
  Gain3 : Gain  Gain=2047
  Quantizer : Quantizer  QuantizationInterval=1
  Quantizer1 : Quantizer  QuantizationInterval=1
  Real-Imag to Complex : RealImagToComplex
  Saturation : Saturate  UpperLimit=2047  LowerLimit=-2048
  Saturation1 : Saturate  UpperLimit=2047  LowerLimit=-2048
  Out : Outport  VectorParamsAs1DForOutWhenUnconnected=off
  wires:
  Real-Imag to Complex/1 -> Out/1
  Gain3/1 -> Complex to Real-Imag/1
  Quantizer1/1 -> Saturation1/1
  Saturation/1 -> Real-Imag to Complex/2
  Saturation1/1 -> Real-Imag to Complex/1
  Complex to Real-Imag/2 -> Quantizer/1
  Complex to Real-Imag/1 -> Quantizer1/1
  Quantizer/1 -> Saturation/1
  In/1 -> Gain3/1

== system adi_ad9361_models/ad9361_rx/LPF_RX/dB2lin ==
  In : Inport
  1/20 : Gain  Gain=1/20
  exp : Math  Operator=10^u  SaturateOnIntegerOverflow=on
  Out : Outport  VectorParamsAs1DForOutWhenUnconnected=off
  wires:
  1/20/1 -> exp/1
  In/1 -> 1/20/1
  exp/1 -> Out/1

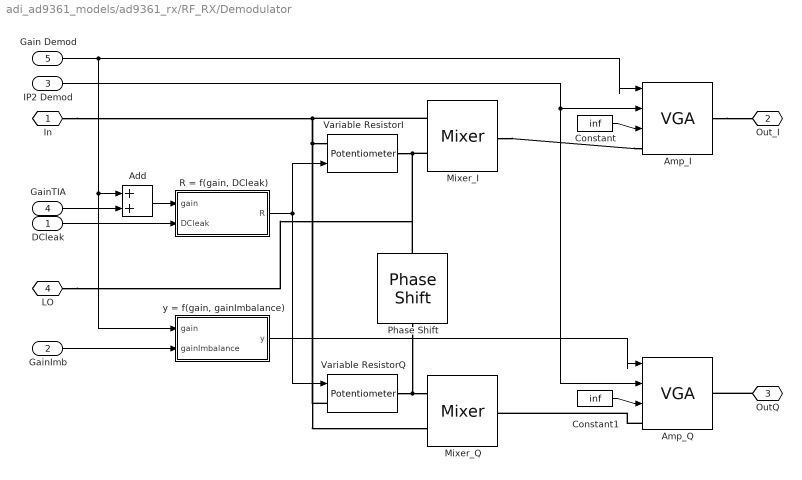
== system adi_ad9361_models/ad9361_rx/RF_RX/Demodulator ==
  DCleak : Inport
  GainImb : Inport  Port=2
  IP2 Demod : Inport  Port=3
  GainTIA : Inport  Port=4
  Gain Demod : Inport  Port=5
  Add : Sum
  Amp_I : simrfV2elements/VGA  classname=vga  Zin=100  Zout=100  IO=Input  InternalGrounding=on
      settings: SourceProductName=RF Blockset  SourceProductBaseCode=RB
  Amp_Q : simrfV2elements/VGA  classname=vga  Zin=100  Zout=100  IO=Input  InternalGrounding=on
      settings: SourceProductName=RF Blockset  SourceProductBaseCode=RB
  Constant : Constant  Value=inf
  Constant1 : Constant  Value=inf
  Mixer_I : simrfV2elements/Mixer  classname=mixer  Source_linear_gain=Available power gain  linear_gain=0 dB  Zin=100  Zout=100  ZLO=inf  Source_Poly=Even and odd order  Poly_Coeffs=[0 1]  IPType=Output  IP2=Inf dBm  IP3=Inf dBm  P1dB=Inf dBm  Psat=Inf dBm  Gcomp=Inf dBm  NF=0  InternalGrounding=on
      settings: SourceProductName=RF Blockset  SourceProductBaseCode=RB
  Mixer_Q : simrfV2elements/Mixer  classname=mixer  Source_linear_gain=Available power gain  linear_gain=0 dB  Zin=100  Zout=100  ZLO=inf  Source_Poly=Even and odd order  Poly_Coeffs=[0 1]  IPType=Output  IP2=Inf dBm  IP3=Inf dBm  P1dB=Inf dBm  Psat=Inf dBm  Gcomp=Inf dBm  NF=0  InternalGrounding=on
      settings: SourceProductName=RF Blockset  SourceProductBaseCode=RB
  Phase Shift : simrfV2elements/Phase Shift  PhaseShift=90 deg  InternalGrounding=on
      settings: SourceProductName=RF Blockset  SourceProductBaseCode=RB
  "R = f(gain, DCleak)" : Subsystem
  Variable ResistorI : simrfV2junction1/Potentiometer  classname=potentiometer  Ron=1e-12 Ohm  Roff=1e12 Ohm  CurveType=Linear  PercentLog=20  PercentAnti=80
      settings: SourceProductName=RF Blockset  SourceProductBaseCode=RB
  Variable ResistorQ : simrfV2junction1/Potentiometer  classname=potentiometer  Ron=1e-12 Ohm  Roff=1e12 Ohm  CurveType=Linear  PercentLog=20  PercentAnti=80
      settings: SourceProductName=RF Blockset  SourceProductBaseCode=RB
  "y = f(gain, gainImbalance)" : Subsystem
  In : PMIOPort  Side=Left
  Out_I : PMIOPort  Port=2  Side=Right
  OutQ : PMIOPort  Port=3  Side=Right
  LO : PMIOPort  Port=4  Side=Left
  wires:
  Constant1/1 -> Amp_Q/3
  Constant/1 -> Amp_I/3
  "y = f(gain, gainImbalance)"/1(y) -> Amp_Q/1
  DCleak/1 -> "R = f(gain, DCleak)"/2(DCleak)
  GainImb/1 -> "y = f(gain, gainImbalance)"/2(gainImbalance)
  Add/1 -> "R = f(gain, DCleak)"/1(gain)
  GainTIA/1 -> Add/2
  "R = f(gain, DCleak)"/1(R) -> Variable ResistorI/1, Variable ResistorQ/1
  IP2 Demod/1 -> Amp_I/2, Amp_Q/2
  Gain Demod/1 -> "y = f(gain, gainImbalance)"/1(gain), Add/1, Amp_I/1
  connections:
  Variable ResistorI/RConn1 -- Phase Shift/LConn1 -- LO/RConn1 -- Mixer_I/LConn2
  Amp_Q/LConn1 -- Mixer_Q/RConn1
  Mixer_I/RConn1 -- Amp_I/LConn1
  OutQ/RConn1 -- Amp_Q/RConn1
  Amp_I/RConn1 -- Out_I/RConn1
  Mixer_I/LConn1 -- Variable ResistorI/LConn1 -- Variable ResistorQ/LConn1 -- Mixer_Q/LConn1 -- In/RConn1
  Variable ResistorQ/RConn1 -- Mixer_Q/LConn2 -- Phase Shift/RConn1
